simulink model "sl_quadrotor"  (R2019b)
settings: Solver=ode45  StartTime=0.0  StopTime=10  MaxStep=0.1  RelTol=1e-3  EnableMultiTasking=on
PreLoadFcn:
  | % load parameters of the default quadrotor
  | disp('Quadrotor parameters loaded by PreLoadFcn')
  | mdl_quadrotor
undefined symbols (not defined in the file or in its folder): rot2
libraries: roblocks x3, simulink x1
settings Model: Creator=corkep  LastModifiedBy=zeyan
settings DataIOCC: LimitDataPoints=on  ReturnWorkspaceOutputs=off
settings OptimizationCC: ExpressionDepthLimit=2147483647  LifeSpan=inf
settings DebuggingCC: UnderspecifiedInitializationDetection=Classic  MergeDetectMultiDrivingBlocksExec=none  SolverPrmCheckMsg=warning  AllowSymbolicDim=off  StateNameClashWarn=warning  SFUnexpectedBacktrackingDiag=warning  SFNoUnconditionalDefaultTransitionDiag=warning  SFExecutionAtInitializationDiag=none  ArithmeticOperatorsInVariantConditions=warning
settings HardwareCC: ProdBitPerPointer=32  ProdBitPerSizeT=32  ProdBitPerPtrDiffT=32  ProdLargestAtomicFloat=None  ProdIntDivRoundTo=Undefined  ProdEndianess=Unspecified  ProdWordSize=32  ProdHWDeviceType=32-bit Generic
settings ModelReferenceCC: PropagateSignalLabelsOutOfModel=off
settings SFSimCC: SimUseLocalCustomCode=off  CustomCodeUndefinedFunction=UseInterfaceOnly
settings RTWCC: RTWUseLocalCustomCode=off
settings CodeAppCC: StateflowObjectComments=on
settings GRTTargetCC: TargetLangStandard=C89/C90 (ANSI)  GeneratePreprocessorConditionals=Disable all  CombineOutputUpdateFcns=off  GRTInterface=on
settings ConfigComp: CovMetricSettings=dw  CovHtmlReporting=on  CovSaveCumulativeToWorkspaceVar=on  CovSaveSingleToWorkspaceVar=on  CovExternalEMLEnable=off  CovSFcnEnable=off

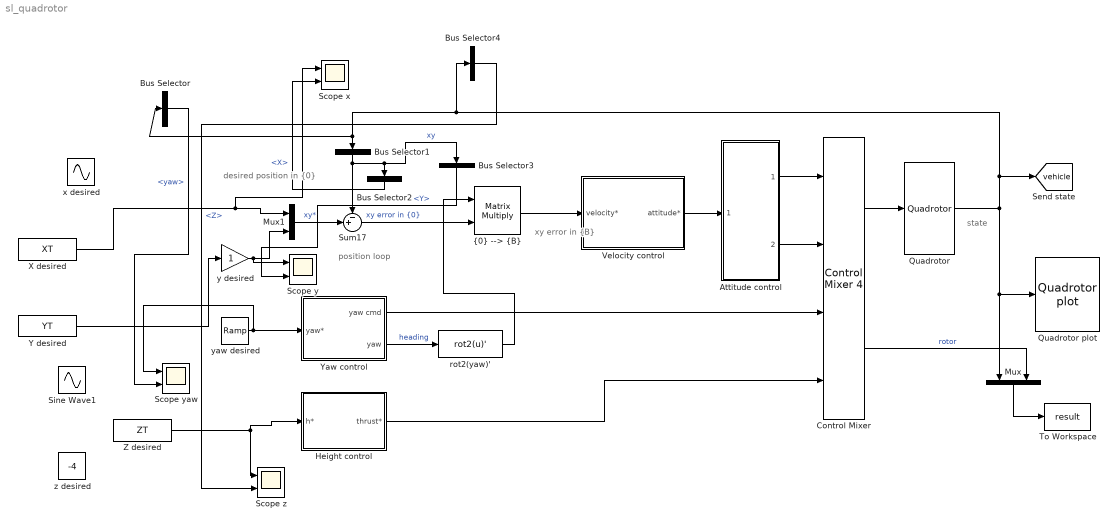
== system sl_quadrotor ==
  note: xy error
      | in {B}
  note: desired position
      | in {0}
  note: position
      | loop
  note: state
  Attitude control : Subsystem  mask{P=100, D=1}
      mask prompts: P "Proportional gain"; D "Derivative gain"
  Bus Selector : BusSelector  OutputSignals=yaw
  Bus Selector1 : BusSelector  OutputSignals=X,Y  OutputAsBus=on
  Bus Selector2 : BusSelector  OutputSignals=X
  Bus Selector3 : BusSelector  OutputSignals=Y
  Bus Selector4 : BusSelector  OutputSignals=Z
  Control Mixer : roblocks/Vehicles/Control Mixer 4  quad=quadrotor  maxrot=1000  minrot=5
  Height control : Subsystem  mask{P=4, D=1, T0=40}
      mask prompts: P "Proportional gain"; D "Derivative gain"; T0 "Thrust feedforward"
  Mux : Mux  Inputs=2
  Mux1 : Mux  Inputs=2
  Quadrotor : roblocks/Vehicles/Quadrotor  quad=quadrotor  x0=[0 0 -0.2]  groundflag=on
  Quadrotor plot : roblocks/Vehicles/Quadrotor plot  quad=quadrotor  xydim=2  zdim=10
  Scope x : Scope  NumInputPorts=2
  Scope y : Scope  NumInputPorts=2
  Scope yaw : Scope  NumInputPorts=2
  Scope z : Scope  NumInputPorts=2
  Sine Wave1 : Sin  Frequency=pi/4  SampleTime=0
  Sum17 : Sum  Inputs=-+|
  To Workspace : ToWorkspace  VariableName=result  SampleTime=-1
  Velocity control : Subsystem  mask{P=0.1, D=2}
      mask prompts: P "Proportional gain"; D "Derivative gain"
  X desired : FromWorkspace  VariableName=XT  SampleTime=0
  Y desired : FromWorkspace  VariableName=YT  SampleTime=0
  Yaw control : Subsystem  mask{P=20, D=2}
      mask prompts: P "Proportional gain"; D "Derivative gain"
  Z desired : FromWorkspace  VariableName=ZT  SampleTime=0
  rot2(yaw)' : MATLABFcn  MATLABFcn=rot2(u)'  OutputDimensions=[2 2]  Output1D=off
  x desired : Sin  Frequency=pi/4  Phase=-pi/2  SampleTime=0
  y desired : Gain
  yaw desired : simulink/Sources/Ramp  slope=0.2  start=1  InitialOutput=0
  z desired : Constant  Value=-4
  "{0} --> {B}" : Product  Multiplication=Matrix(*)  RndMeth=Zero
  tag scope: vehicle=global
  wires:
  Quadrotor/1 -> Quadrotor plot/1, Mux/1, [vehicle], Bus Selector4/1, Bus Selector/1, Bus Selector1/1
  X desired/1 -> Scope x/1, Mux1/1
  Y desired/1 -> y desired/1
  Mux/1 -> To Workspace/1
  Control Mixer/2 -> Mux/2  "rotor"
  Sum17/1 -> "{0} --> {B}"/2  "xy error in {0}"
  "{0} --> {B}"/1 -> Velocity control/1(velocity*)
  Velocity control/1(attitude*) -> Attitude control/1(attitude*)
  Yaw control/2(yaw) -> rot2(yaw)'/1  "heading"
  Yaw control/1(yaw cmd) -> Control Mixer/3
  yaw desired/1 -> Scope yaw/1, Yaw control/1(yaw*)
  Z desired/1 -> Height control/1(h*), Scope z/1
  Mux1/1 -> Sum17/2  "xy*"
  Bus Selector1/1 -> Bus Selector3/1, Bus Selector2/1, Sum17/1  "xy"
  rot2(yaw)'/1 -> "{0} --> {B}"/1
  Attitude control/1(roll torque*) -> Control Mixer/1
  Attitude control/2(pitch torque*) -> Control Mixer/2
  Control Mixer/1 -> Quadrotor/1
  Height control/1(thrust*) -> Control Mixer/4
  Bus Selector2/1 -> Scope x/2  "<X>"
  y desired/1 -> Scope y/1, Mux1/2
  Bus Selector3/1 -> Scope y/2  "<Y>"
  Bus Selector/1 -> Scope yaw/2  "<yaw>"
  Bus Selector4/1 -> Scope z/2  "<Z>"

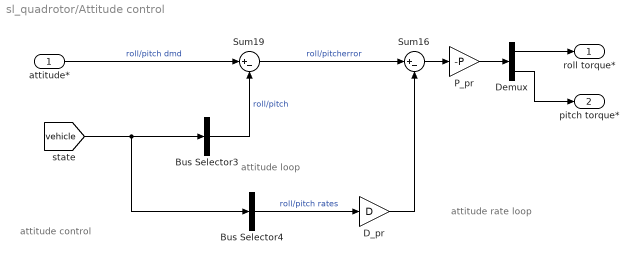
== system sl_quadrotor/Attitude control ==
  note: attitude control
  note: attitude rate loop
  note: attitude loop
  attitude* : Inport
  Bus Selector3 : BusSelector  OutputSignals=roll,pitch  OutputAsBus=on
  Bus Selector4 : BusSelector  OutputSignals=droll,dpitch  OutputAsBus=on
  D_pr : Gain  Gain=D
  Demux : Demux  Outputs=2
  P_pr : Gain  Gain=-P
  Sum16 : Sum  Inputs=|+-
  Sum19 : Sum  Inputs=|+-
  roll torque* : Outport
  pitch torque* : Outport  Port=2
  wires:
  [vehicle] -> Bus Selector4/1, Bus Selector3/1
  attitude*/1 -> Sum19/1  "roll/pitch dmd"
  Bus Selector3/1 -> Sum19/2  "roll/pitch"
  Bus Selector4/1 -> D_pr/1  "roll/pitch rates"
  Sum19/1 -> Sum16/1  "roll/pitcherror"
  Sum16/1 -> P_pr/1
  P_pr/1 -> Demux/1
  D_pr/1 -> Sum16/2
  Demux/2 -> pitch torque*/1
  Demux/1 -> roll torque*/1

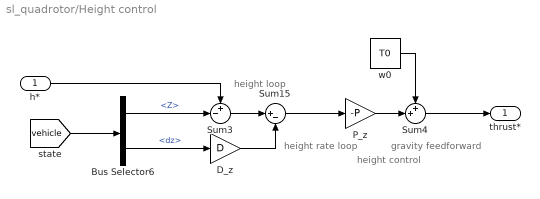
== system sl_quadrotor/Height control ==
  note: height control
  note: gravity feedforward
  note: height rate
      | loop
  note: height
      | loop
  h* : Inport
  Bus Selector6 : BusSelector  OutputSignals=Z,dz
  D_z : Gain  Gain=D
  P_z : Gain  Gain=-P
  Sum15 : Sum  Inputs=|+-
  Sum3 : Sum  Inputs=+-|
  Sum4 : Sum  Inputs=++|
  w0 : Constant  Value=T0  SampleTime=0
  thrust* : Outport
  wires:
  w0/1 -> Sum4/1
  Sum15/1 -> P_z/1
  P_z/1 -> Sum4/2
  Bus Selector6/1 -> Sum3/2  "<Z>"
  h*/1 -> Sum3/1
  Sum3/1 -> Sum15/1
  Bus Selector6/2 -> D_z/1  "<dz>"
  D_z/1 -> Sum15/2
  Sum4/1 -> thrust*/1
  [vehicle] -> Bus Selector6/1

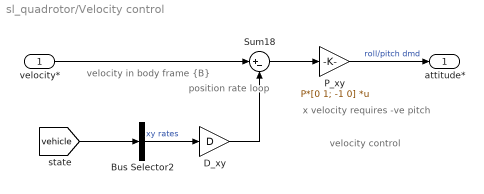
== system sl_quadrotor/Velocity control ==
  note: x velocity requires -ve pitch
  note: velocity in body frame {B}
  note: velocity control
  note: position rate
      | loop
  velocity* : Inport
  Bus Selector2 : BusSelector  OutputSignals=dx,dy  OutputAsBus=on
  D_xy : Gain  Gain=D
  P_xy : Gain  Gain=P*[0 1; -1 0]  Multiplication=Matrix(K*u)
  Sum18 : Sum  Inputs=|+-
  attitude* : Outport
  wires:
  Bus Selector2/1 -> D_xy/1  "xy rates"
  D_xy/1 -> Sum18/2
  Sum18/1 -> P_xy/1
  velocity*/1 -> Sum18/1
  [vehicle] -> Bus Selector2/1
  P_xy/1 -> attitude*/1  "roll/pitch dmd"

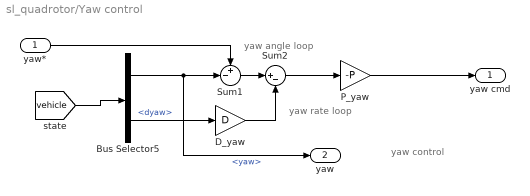
== system sl_quadrotor/Yaw control ==
  note: yaw control
  note: yaw rate
      | loop
  note: yaw angle
      | loop
  yaw* : Inport
  Bus Selector5 : BusSelector  OutputSignals=yaw,dyaw
  D_yaw : Gain  Gain=D
  P_yaw : Gain  Gain=-P
  Sum1 : Sum  Inputs=+-|
  Sum2 : Sum  Inputs=|+-
  yaw cmd : Outport
  yaw : Outport  Port=2
  wires:
  [vehicle] -> Bus Selector5/1
  P_yaw/1 -> yaw cmd/1
  Bus Selector5/1 -> yaw/1, Sum1/2  "<yaw>"
  Sum2/1 -> P_yaw/1
  Bus Selector5/2 -> D_yaw/1  "<dyaw>"
  D_yaw/1 -> Sum2/2
  Sum1/1 -> Sum2/1
  yaw*/1 -> Sum1/1
